simulink model "bspline_polytraj_ex1"  (R2020a)
settings: Solver=VariableStepAuto  StartTime=0.0  StopTime=140.00  RelTol=1e-3
undefined symbols (not defined in the file or in its folder): B, eul2tform, Spline, trvec2tform, waypoints, wpts
libraries: robotcorelib x3, simulink x3
settings Model: Creator=The MathWorks, Inc.  LastModifiedBy=Lamarre
settings SFSimCC: CustomCodeUndefinedFunction=UseInterfaceOnly

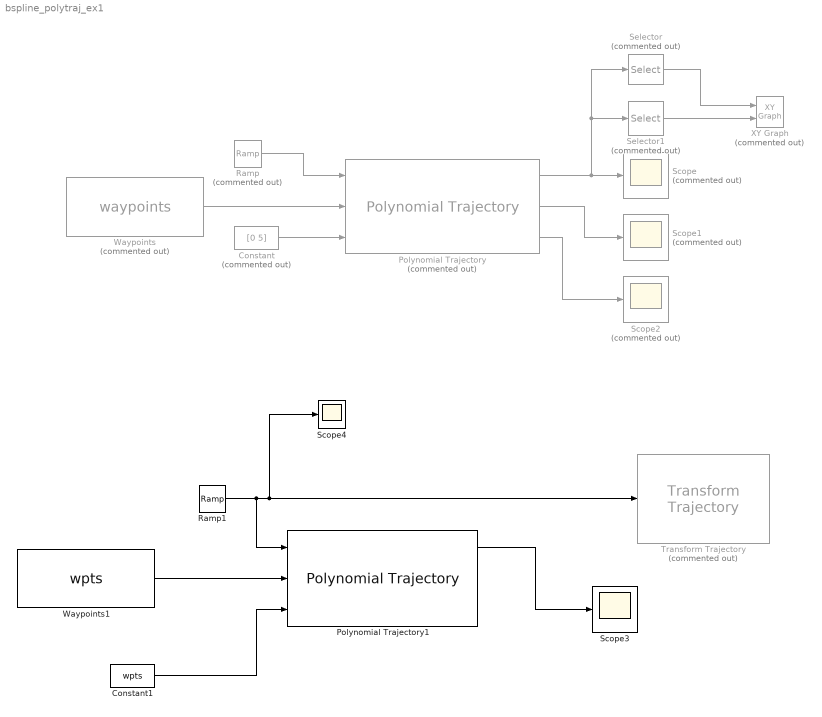
== system bspline_polytraj_ex1 ==
  Constant : Constant  Commented=on  Value=[0 5]
  Constant1 : Constant  Value=wpts
  Polynomial Trajectory : robotcorelib/Polynomial Trajectory  Commented=on  WaypointSource=External  Waypoints=wayPoints  TimePoints=[ 0, 1, 2, 3, 4 ]  TimeInterval=[0,5]  Method=B-Spline  ParameterSource=Internal  VelocityBoundaryCondition=zeros( 2, 5 )  AccelerationBoundaryCondition=zeros( 2, 5 )  SimulateUsing=Interpreted execution
      settings: SourceProductBaseCode=NV,RO,RR
  Polynomial Trajectory1 : robotcorelib/Polynomial Trajectory  WaypointSource=External  Waypoints=[ 0, 2, 1, 5, 0; -1, 3, 1, 4, 4 ]  TimePoints=[ 0, 1, 2, 3, 4 ]  TimeInterval=[ 1, 4 ]  Method=Cubic Polynomial  ParameterSource=Internal  VelocityBoundaryCondition=zeros(3,10)  AccelerationBoundaryCondition=zeros( 2, 5 )  SimulateUsing=Interpreted execution
      settings: SourceProductBaseCode=NV,RO,RR
  Ramp : simulink/Sources/Ramp  Commented=on  slope=1  start=0  InitialOutput=0
  Ramp1 : simulink/Sources/Ramp  slope=1  start=0  InitialOutput=0
  Scope : Scope  Commented=on
  Scope1 : Scope  Commented=on
  Scope2 : Scope  Commented=on
  Scope3 : Scope
  Scope4 : Scope
  Selector : Selector  Commented=on  InputPortWidth=2  IndexOptions=Index vector (dialog)  Indices=1  OutputSizes=1
  Selector1 : Selector  Commented=on  InputPortWidth=2  IndexOptions=Index vector (dialog)  Indices=2  OutputSizes=1
  Transform Trajectory : robotcorelib/Transform Trajectory  Commented=on  WaypointSource=Internal  T0=trvec2tform( [ 1, 10, -1 ] )  TF=eul2tform( [ 0, pi, pi / 2 ] )  TimeInterval=[ 2, 3 ]  CustomTimeScaling=off  ParameterSource=Internal  TSTime=2:0.1:3  TimeScaling=[ 0:0.1:1; ones( 1, 11 ); zeros( 1, 11 ) ]  SimulateUsing=Interpreted execution
      settings: SourceProductBaseCode=NV,RO,RR
  Waypoints : Constant  Commented=on  Value=waypoints
  Waypoints1 : Constant  Value=wpts
  XY Graph : simulink/Sinks/XY Graph  Commented=on  xmin=-3  xmax=5  ymin=-1  ymax=5  st=-1
  wires:
  Ramp/1 -> Polynomial Trajectory/1
  Polynomial Trajectory/1 -> Selector1/1, Selector/1, Scope/1
  Polynomial Trajectory/2 -> Scope1/1
  Polynomial Trajectory/3 -> Scope2/1
  Selector1/1 -> XY Graph/2
  Selector/1 -> XY Graph/1
  Constant/1 -> Polynomial Trajectory/3
  Waypoints/1 -> Polynomial Trajectory/2
  Ramp1/1 -> Polynomial Trajectory1/1, Scope4/1, Transform Trajectory/1
  Waypoints1/1 -> Polynomial Trajectory1/2
  Constant1/1 -> Polynomial Trajectory1/3
  Polynomial Trajectory1/1 -> Scope3/1
